simulink model "odqsim_fboq"  (R2012b)
settings: Solver=FixedStepDiscrete  SolverMode=SingleTasking  StartTime=0.0  StopTime=10.0  FixedStep=Ts  RelTol=1e-3
values from neighbouring files (symbols this model uses):
  K = odqdata.K    [odqlab_interact.m]
  P = odqdata.P    [odqlab_interact.m]
  Q = odqanly(G)    [odq.m]    (also in odqlab_interact.m = odqdata.Q; odqlab_verify.m = odqdata.Q; odqreal.m = orderfields(Q); odqsim.m = varargin{2})
undefined symbols (not defined in the file or in its folder): Ts
libraries: odqblock x5
settings Model: CovMetricSettings=dwe  CovHtmlReporting=off  covSaveCumulativeToWorkspaceVar=off  CovSaveSingleToWorkspaceVar=off  CovExternalEMLEnable=on  Creator=morita  LastModifiedBy=morita
settings DataIOCC: LimitDataPoints=off  SaveFormat=StructureWithTime
settings OptimizationCC: ExpressionDepthLimit=128
settings DebuggingCC: UnderspecifiedInitializationDetection=Simplified  MergeDetectMultiDrivingBlocksExec=error  SolverPrmCheckMsg=none  FrameProcessingCompatibilityMsg=error  StateNameClashWarn=none  SFUnexpectedBacktrackingDiag=error  SFNoUnconditionalDefaultTransitionDiag=error
settings HardwareCC: ProdBitPerPointer=64  ProdLargestAtomicFloat=Float  ProdIntDivRoundTo=Zero  ProdEndianess=LittleEndian  ProdHWDeviceType=Specified
settings ModelReferenceCC: PropagateSignalLabelsOutOfModel=on
settings CodeAppCC: CustomSymbolStrType=$N$R$M_T
settings GRTTargetCC: CodeReplacementLibrary=C99 (ISO)  GeneratePreprocessorConditionals=Use local settings

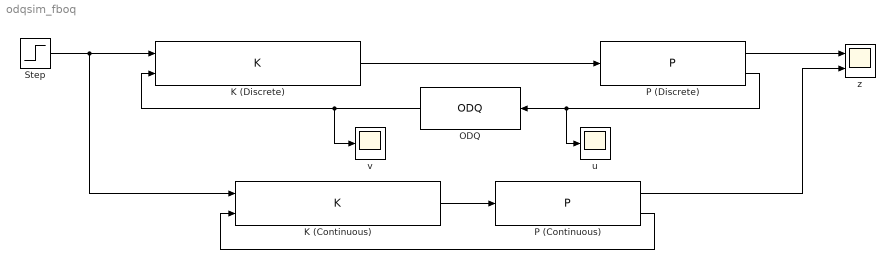
== system odqsim_fboq ==
  K (Continuous) : odqblock/K  A=K.a  B1=K.b1  B2=K.b2  C=K.c  D1=K.d1  D2=K.d2  Ts=Ts  x0=x0
  K (Discrete) : odqblock/K  A=K.a  B1=K.b1  B2=K.b2  C=K.c  D1=K.d1  D2=K.d2  Ts=Ts  x0=x0
  ODQ : odqblock/ODQ  A=Q.a  B1=Q.b1  B2=Q.b2  C=Q.c  d=d  Ts=Ts
  P (Continuous) : odqblock/P  A=P.a  B=P.b  C1=P.c1  C2=P.c2  Ts=Ts  x0=x0
  P (Discrete) : odqblock/P  A=P.a  B=P.b  C1=P.c1  C2=P.c2  Ts=Ts  x0=x0
  Step : Step  Time=0  SampleTime=0
  u : Scope
      settings: TimeRange=auto  LimitDataPoints=on  MaxDataPoints=5000  SaveToWorkspace=off  SaveName=ScopeData4  YMin=-10  YMax=10  SampleTime=-1  DataFormat=Array
  v : Scope
      settings: TimeRange=auto  LimitDataPoints=on  MaxDataPoints=5000  SaveToWorkspace=off  YMin=-10  YMax=10  SampleTime=-1  DataFormat=Array
  z : Scope  NumInputPorts=2
      settings: TimeRange=auto  MaxDataPoints=5000  SaveToWorkspace=off  SaveName=ScopeData  YMin=-10~-5  YMax=10~5  SampleTime=-1
  wires:
  K (Continuous)/1 -> P (Continuous)/1
  K (Discrete)/1 -> P (Discrete)/1
  P (Continuous)/2 -> K (Continuous)/2
  P (Continuous)/1 -> z/2
  P (Discrete)/2 -> u/1, ODQ/1
  Step/1 -> K (Continuous)/1, K (Discrete)/1
  P (Discrete)/1 -> z/1
  ODQ/1 -> v/1, K (Discrete)/2
